simulink model "LT_AE220"  (R2025b)
settings: Solver=FixedStepAuto  StartTime=0.0  StopTime=inf  FixedStep=1E-2  RelTol=1e-3
libraries: aerolibanimutils x1
settings Model: Creator=abstract  LastModifiedBy=abstract

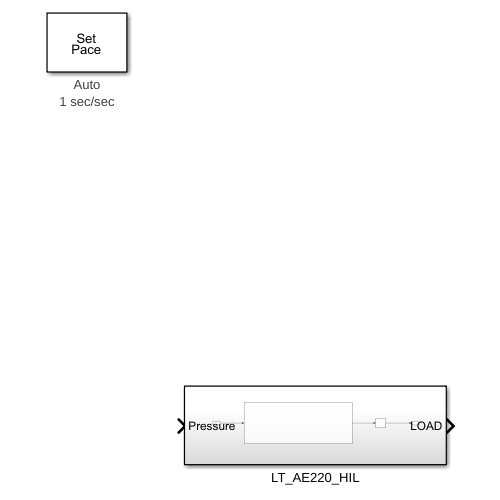
[thumbnail: Simulink's stored preview of the top-level diagram]
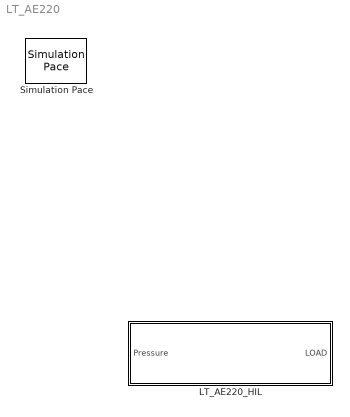
== system LT_AE220 ==
  LT_AE220_HIL : Subsystem
  Simulation Pace : aerolibanimutils/Simulation Pace  SimulationPace=1  SleepMode=Auto  OutputPaceError=off  SampleTime=-1

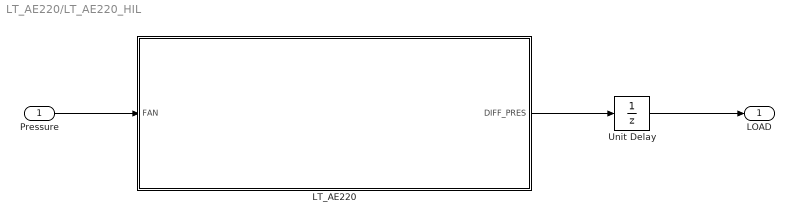
== system LT_AE220/LT_AE220_HIL ==
  Pressure : Inport  OutDataTypeStr=single
  LT_AE220 : MATLAB Function  TreatAsAtomicUnit=on
  Unit Delay : UnitDelay  SampleTime=-1  HasFrameUpgradeWarning=on
  LOAD : Outport  OutDataTypeStr=single
  wires:
  Pressure/1 -> LT_AE220/1(FAN)
  Unit Delay/1 -> LOAD/1
  LT_AE220/1(DIFF_PRES) -> Unit Delay/1

== matlab function LT_AE220/LT_AE220_HIL/LT_AE220 ==
  data: FAN input; DIFF_PRES output
function DIFF_PRES = LT_AE220(FAN)

DIFF_PRES = Get_WT_State();
